simulink model "d5_model_deneme"  (R2014a)
settings: Solver=FixedStepDiscrete  StartTime=0.0  StopTime=1.0  FixedStep=0.001  RelTol=1e-3
settings Model: Creator=cya  LastModifiedBy=cya

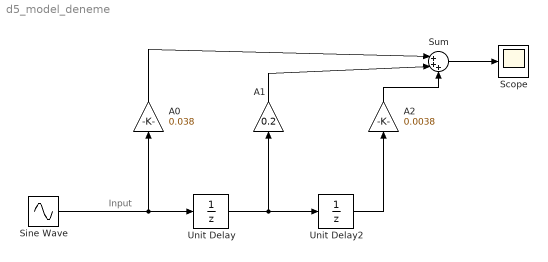
== system d5_model_deneme ==
  note: Input
  A0 : Gain  Gain=0.038
  A1 : Gain  Gain=0.2
  A2 : Gain  Gain=0.0038
  Scope : Scope
      settings: TimeRange=1  YMin=0  YMax=0.0018
  Sine Wave : Sin  Frequency=1200  SampleTime=0
  Sum : Sum  Inputs=|+++
  Unit Delay : UnitDelay  SampleTime=-1
  Unit Delay2 : UnitDelay  SampleTime=-1
  wires:
  Unit Delay/1 -> Unit Delay2/1, A1/1
  Sine Wave/1 -> A0/1, Unit Delay/1
  Unit Delay2/1 -> A2/1
  A1/1 -> Sum/2
  A0/1 -> Sum/1
  A2/1 -> Sum/3
  Sum/1 -> Scope/1
